simulink model "CLSfixed_pace"  (R2024b)
settings: Solver=FixedStepAuto  StartTime=0.0  StopTime=stoptime  FixedStep=stepsize  RelTol=1e-3
undefined symbols (not defined in the file or in its folder): AVI, cfg_length, LCP_delay, LRI, pNode_length, pPath_length, PVARP, stepsize, URI, VRP
libraries: Libs_unified x157
(part 1 of 3)
settings Model: SimulationMode=accelerator  PacingRate=0.001000  Creator=ball907  LastModifiedBy=ball907

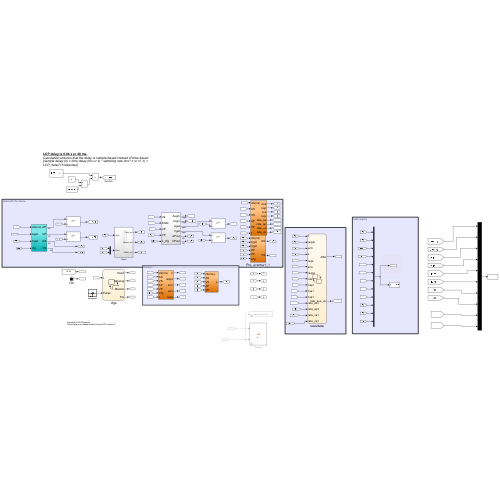
[thumbnail: Simulink's stored preview of the top-level diagram]
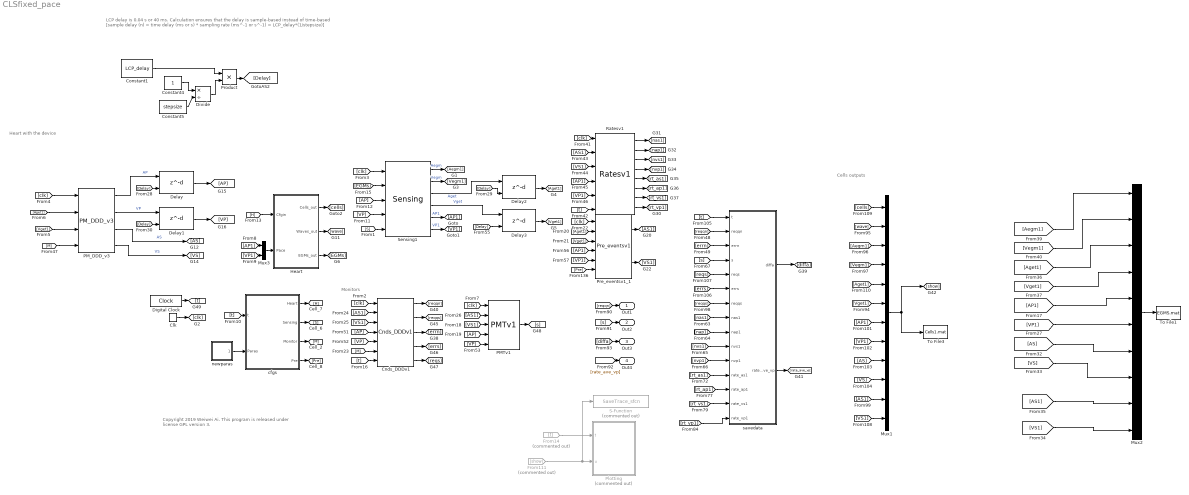
== system CLSfixed_pace ==
  note: Cells outputs
  note: Copyright 2019 Weiwei Ai.
      | This program is released under license GPL version 3.
  note: Heart with the device
  note: Monitors
  note: LCP delay is 0.04 s or 40 ms.
      | Calculation ensures that the delay is sample-based instead of time-based
      | [sample delay (n) = time delay (ms or s) * sampling rate (ms^-1 or s^-1) = LCP_delay*(1/stepsize)]
  Clk : DiscretePulseGenerator  PulseType=Time based  Period=1  PulseWidth=100*stepsize
  Cnds_DDDv1 : Libs_unified/Cnds_DDDv1  SystemSampleTime=-1  VariantActivationTime=update diagram  AllowFlexibleInterface=on  Latency=0  AutoFrameSizeCalculation=off
  Constant1 : Constant  Value=LCP_delay
  Constant4 : Constant
  Constant5 : Constant  Value=stepsize
  Delay{,1..3} (4 alike) : Delay  DelayLengthSource=Input port  DelayLengthUpperLimit=10000
      settings: InputPortMap=u0,p1
  Digital Clock : DigitalClock  SampleTime=stepsize
  Divide : Product  Inputs=*/
  From111 : From  Commented=on  GotoTag=show
  From14 : From  Commented=on  GotoTag=t
  Heart : Subsystem
  Mux1 : Mux  Inputs=12
  Mux2 : Mux  Inputs=10
  Mux3 : Mux  Inputs=2
  PMTv1 : Libs_unified/PMTv1  SystemSampleTime=-1  VariantActivationTime=update diagram  AllowFlexibleInterface=on  Latency=0  AutoFrameSizeCalculation=off
  PM_DDD_v3 : Libs_unified/PM_DDD_v3  SystemSampleTime=-1  VariantActivationTime=update diagram  AllowFlexibleInterface=on  Latency=0  AutoFrameSizeCalculation=off
  Plotting : MATLAB Function  Commented=on  TreatAsAtomicUnit=on  SystemSampleTime=stepsize*5
  Pre_eventsv1_1 : Libs_unified/Pre_eventsv1  SystemSampleTime=-1  VariantActivationTime=update diagram  AllowFlexibleInterface=on  Latency=0  AutoFrameSizeCalculation=off
  Product : Product
  Ratesv1 : Libs_unified/Ratesv1  SystemSampleTime=-1  VariantActivationTime=update diagram  AllowFlexibleInterface=on  Latency=0  AutoFrameSizeCalculation=off
  S-Function : S-Function  Commented=on  FunctionName=SaveTrace_sfcn  Parameters=1  SFunctionDeploymentMode=off  EnableBusSupport=off
  Sensing1 : Libs_unified/Sensing  SystemSampleTime=-1  VariantActivationTime=update diagram  AllowFlexibleInterface=on  Latency=0  AutoFrameSizeCalculation=off
  To File1 : ToFile  Filename=EGMS.mat  MatrixName=pacing
      settings: Decimation=2
  To File3 : ToFile  Filename=Cells1.mat  MatrixName=cells
      settings: Decimation=2
  cfgs : Stateflow chart  TreatAsAtomicUnit=on
  newparas : MATLAB Function  TreatAsAtomicUnit=on
  savedata : Stateflow chart  TreatAsAtomicUnit=on
  Out1 : Outport
  Out2 : Outport  Port=2
  Out3 : Outport  Port=3
  Out4 : Outport  Port=4
  wires:
  Ratesv1/4 -> [nvp1]
  [reqqn] -> Out1/1
  [AS1] -> Ratesv1/2
  Sensing1/1 -> [Aegm1]  "Aegm"
  [AP1] -> Mux1/7
  [rt_as1] -> savedata/12(rate_as1)
  Ratesv1/3 -> [nvs1]
  [reqs] -> savedata/5(reqs)
  [t] -> Ratesv1/6
  Ratesv1/2 -> [nap1]
  [AS1] -> Cnds_DDDv1/2
  [AS] -> Mux1/9
  [AS1] -> PMTv1/2
  [M] -> PM_DDD_v3/4
  [s] -> Out2/1
  [VP1] -> Ratesv1/5
  [AP1] -> Mux3/1
  [VP1] -> Pre_eventsv1_1/5
  [t] -> savedata/1(t)
  savedata/1(diffa) -> [diffa]
  Cnds_DDDv1/1 -> [reqqn]
  [AP1] -> Ratesv1/4
  [nap1] -> savedata/9(nap1)
  Sensing1/6 -> [VP1]  "VP1"
  Sensing1/5 -> [AP1]  "AP1"
  PMTv1/1 -> [s]
  [M] -> Cnds_DDDv1/6
  [AP1] -> Pre_eventsv1_1/4
  [s] -> savedata/4(s)
  Heart/3(EGMs_out) -> [EGMs]
  [diffa] -> Out3/1
  [cells] -> Mux1/1
  Cnds_DDDv1/4 -> [errs]
  Ratesv1/7 -> [rt_vs1]
  [clk] -> PM_DDD_v3/1
  Pre_eventsv1_1/1 -> [AS1]
  [Vget1] -> Mux1/6
  [VP1] -> Mux1/8
  [VS1] -> Cnds_DDDv1/3
  [clk] -> Sensing1/1
  Ratesv1/6 -> [rt_ap1]
  [S] -> Sensing1/5
  Digital Clock/1 -> [t]
  [AP] -> PMTv1/4
  [nas1] -> savedata/8(nas1)
  [reqqn] -> savedata/2(reqqn)
  Clk/1 -> [clk]
  [VS] -> Mux1/10
  [nvp1] -> savedata/11(nvp1)
  Cnds_DDDv1/3 -> [errn]
  Ratesv1/5 -> [rt_as1]
  Sensing1/2 -> [Vegm1]  "Vegm"
  [H] -> Heart/1(Cfgin)
  Cnds_DDDv1/2 -> [reqqs]
  [VS1] -> PMTv1/3
  [AS1] -> Mux1/11
  [Aget1] -> Pre_eventsv1_1/2
  [errs] -> savedata/6(errs)
  [clk] -> PMTv1/1
  Pre_eventsv1_1/2 -> [VS1]
  [rt_vp1] -> savedata/15(rate_vp1)
  [VS1] -> Mux1/12
  Ratesv1/1 -> [nas1]
  [VP] -> PMTv1/5
  [clk] -> Ratesv1/1
  PM_DDD_v3/4 -> [VS]  "VS"
  savedata/2(rate_ave_vp) -> [rate_ave_vp]
  [rt_ap1] -> savedata/13(rate_ap1)
  [Aegm1] -> Mux1/3
  [t] -> Cnds_DDDv1/7
  [reqqs] -> savedata/7(reqqs)
  [rate_ave_vp] -> Out4/1
  Cnds_DDDv1/5 -> [reqs]
  [VP] -> Cnds_DDDv1/5
  [VP1] -> Mux3/2
  Mux3/1 -> Heart/2(Pace)
  [clk] -> Pre_eventsv1_1/1
  Heart/1(Cells_out) -> [cells]
  [errn] -> savedata/3(errn)
  [rt_vs1] -> savedata/14(rate_vs1)
  [Aget1] -> Mux1/5
  [Pre] -> Pre_eventsv1_1/6
  [VS1] -> Ratesv1/3
  Mux1/1 -> [show], To File3/1
  [nvs1] -> savedata/10(nvs1)
  [Vget1] -> Pre_eventsv1_1/3
  [Vegm1] -> Mux1/4
  [AP] -> Cnds_DDDv1/4
  Heart/2(Waves_out) -> [wave]
  [wave] -> Mux1/2
  Ratesv1/8 -> [rt_vp1]
  [clk] -> Cnds_DDDv1/1
  cfgs/2(Sensing) -> [S]
  cfgs/4(Pre) -> [Pre]
  newparas/1(newparas) -> cfgs/2(Paras)
  cfgs/3(Monitor) -> [M]
  cfgs/1(Heart) -> [H]
  [t] -> cfgs/1(t)
  From111/1 -> S-Function/1, Plotting/2(u)
  From14/1 -> Plotting/1(t)
  PM_DDD_v3/2 -> Delay1/1  "VP"
  PM_DDD_v3/3 -> [AS]  "AS"
  [VS] -> Mux2/8
  [AS] -> Mux2/7
  [Vegm1] -> Mux2/2
  [Aegm1] -> Mux2/1
  Mux2/1 -> To File1/1
  [Aget1] -> Mux2/3
  [Vget1] -> Mux2/4
  [AP1] -> Mux2/5
  [VP1] -> Mux2/6
  [AS1] -> Mux2/9
  [VS1] -> Mux2/10
  PM_DDD_v3/1 -> Delay/1  "AP"
  [EGMs] -> Sensing1/2
  [AP] -> Sensing1/3
  [VP] -> Sensing1/4
  [Aget1] -> PM_DDD_v3/2
  [Vget1] -> PM_DDD_v3/3
  Delay1/1 -> [VP]
  Delay/1 -> [AP]
  Sensing1/3 -> Delay2/1  "Aget"
  Delay2/1 -> [Aget1]
  Delay3/1 -> [Vget1]
  Sensing1/4 -> Delay3/1  "Vget"
  Product/1 -> [Delay]
  Divide/1 -> Product/2
  [Delay] -> Delay/2
  Constant4/1 -> Divide/1
  Constant5/1 -> Divide/2
  [Delay] -> Delay1/2
  [Delay] -> Delay2/2
  [Delay] -> Delay3/2
  Constant1/1 -> Product/1
